simulink model "tanque"  (R2020b)
settings: Solver=ode3  StartTime=0.0  StopTime=5000  FixedStep=0.1  RelTol=1e-3
libraries: simulink x1
settings Model: Creator=Darkhorrow  LastModifiedBy=Darkhorrow

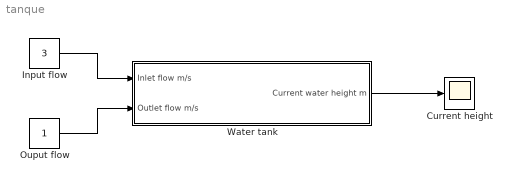
== system tanque ==
  Current height : Scope
  Input flow : Constant  Value=3
  Ouput flow : Constant
  Water tank : Subsystem
  wires:
  Input flow/1 -> Water tank/1(Inlet flow m/s)
  Ouput flow/1 -> Water tank/2(" Outlet flow m/s")
  Water tank/1(Current water height m) -> Current height/1

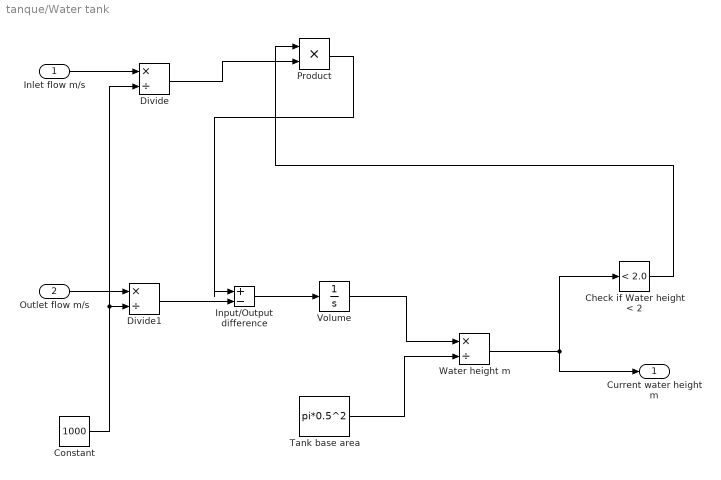
== system tanque/Water tank ==
  Inlet flow m/s : Inport
  " Outlet flow m/s" : Inport  Port=2
  "Check if Water height < 2 " : simulink/Logic and Bit Operations/Compare To Constant  relop=<  const=2.0  OutDataTypeStr=uint8
  Constant : Constant  Value=1000
  Divide : Product  Inputs=*/
  Divide1 : Product  Inputs=*/
  Input/Output difference : Sum  Inputs=|+-
  Product : Product
  Tank base area : Constant  Value=pi*0.5^2
  Volume : Integrator
  Water height m : Product  Inputs=*/
  Current water height m : Outport
  wires:
  " Outlet flow m/s"/1 -> Divide1/1
  Tank base area/1 -> Water height m/2
  Water height m/1 -> Current water height m/1, "Check if Water height < 2 "/1
  Divide1/1 -> Input/Output difference/2
  Inlet flow m/s/1 -> Divide/1
  Volume/1 -> Water height m/1
  Constant/1 -> Divide1/2, Divide/2
  Product/1 -> Input/Output difference/1
  Input/Output difference/1 -> Volume/1
  Divide/1 -> Product/2
  "Check if Water height < 2 "/1 -> Product/1
